simulink library "mDataStoreBlocks_library"  (R2013b)
settings: Solver=ode45  StartTime=0.0  StopTime=10.0  RelTol=1e-3
settings Model: Creator=hungdang  LastModifiedBy=hungdang

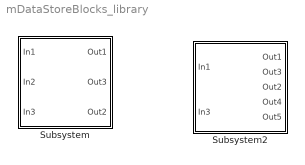
== system mDataStoreBlocks_library ==
  Subsystem : Subsystem  TreatAsAtomicUnit=on
  Subsystem2 : Subsystem  TreatAsAtomicUnit=on
      mask help: This is a simple mask.

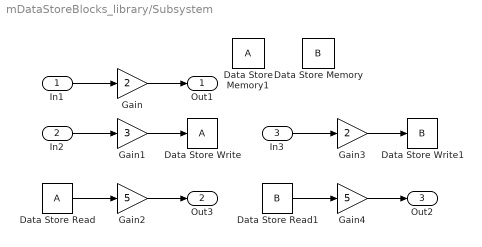
== system mDataStoreBlocks_library/Subsystem ==
  In1 : Inport
  In2 : Inport  Port=2
  In3 : Inport  Port=3
  Data Store Memory : DataStoreMemory  DataStoreName=B  ReadBeforeWriteMsg=warning  WriteAfterWriteMsg=warning  WriteAfterReadMsg=warning
  Data Store Memory1 : DataStoreMemory  ReadBeforeWriteMsg=warning  WriteAfterWriteMsg=warning  WriteAfterReadMsg=warning
  Data Store Read : DataStoreRead
  Data Store Read1 : DataStoreRead  DataStoreName=B
  Data Store Write : DataStoreWrite
  Data Store Write1 : DataStoreWrite  DataStoreName=B
  Gain : Gain  Gain=2
  Gain1 : Gain  Gain=3
  Gain2 : Gain  Gain=5
  Gain3 : Gain  Gain=2
  Gain4 : Gain  Gain=5
  Out1 : Outport
  Out3 : Outport  Port=2
  Out2 : Outport  Port=3
  wires:
  Gain/1 -> Out1/1
  In1/1 -> Gain/1
  Gain1/1 -> Data Store Write/1
  In2/1 -> Gain1/1
  Data Store Read/1 -> Gain2/1
  Gain2/1 -> Out3/1
  Gain3/1 -> Data Store Write1/1
  In3/1 -> Gain3/1
  Data Store Read1/1 -> Gain4/1
  Gain4/1 -> Out2/1

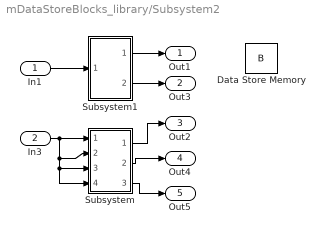
== system mDataStoreBlocks_library/Subsystem2 ==
  In1 : Inport
  In3 : Inport  Port=2
  Data Store Memory : DataStoreMemory  DataStoreName=B  ReadBeforeWriteMsg=warning  WriteAfterWriteMsg=warning  WriteAfterReadMsg=warning
  Subsystem : Subsystem
  Subsystem1 : Subsystem
  Out1 : Outport
  Out3 : Outport  Port=2
  Out2 : Outport  Port=3
  Out4 : Outport  Port=4
  Out5 : Outport  Port=5
  wires:
  Subsystem/3(Out3) -> Out5/1
  Subsystem/2(Out1) -> Out4/1
  Subsystem1/2(Out3) -> Out3/1
  Subsystem1/1(Out1) -> Out1/1
  In1/1 -> Subsystem1/1(In1)
  Subsystem/1(Out2) -> Out2/1
  In3/1 -> Subsystem/1(In3), Subsystem/3(In2), Subsystem/4(In4), Subsystem/2(In1)

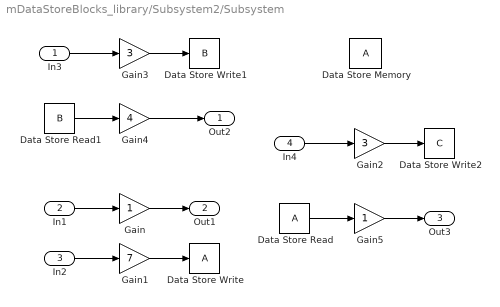
== system mDataStoreBlocks_library/Subsystem2/Subsystem ==
  In3 : Inport
  In1 : Inport  Port=2
  In2 : Inport  Port=3
  In4 : Inport  Port=4
  Data Store Memory : DataStoreMemory  ReadBeforeWriteMsg=warning  WriteAfterWriteMsg=warning  WriteAfterReadMsg=warning
  Data Store Read : DataStoreRead
  Data Store Read1 : DataStoreRead  DataStoreName=B
  Data Store Write : DataStoreWrite
  Data Store Write1 : DataStoreWrite  DataStoreName=B
  Data Store Write2 : DataStoreWrite  DataStoreName=C
  Gain : Gain
  Gain1 : Gain  Gain=7
  Gain2 : Gain  Gain=3
  Gain3 : Gain  Gain=3
  Gain4 : Gain  Gain=4
  Gain5 : Gain
  Out2 : Outport
  Out1 : Outport  Port=2
  Out3 : Outport  Port=3
  wires:
  Gain2/1 -> Data Store Write2/1
  In4/1 -> Gain2/1
  Gain5/1 -> Out3/1
  Data Store Read/1 -> Gain5/1
  In2/1 -> Gain1/1
  Gain1/1 -> Data Store Write/1
  In1/1 -> Gain/1
  Gain/1 -> Out1/1
  Gain3/1 -> Data Store Write1/1
  Data Store Read1/1 -> Gain4/1
  Gain4/1 -> Out2/1
  In3/1 -> Gain3/1

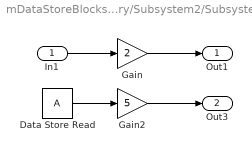
== system mDataStoreBlocks_library/Subsystem2/Subsystem1 ==
  In1 : Inport
  Data Store Read : DataStoreRead
  Gain : Gain  Gain=2
  Gain2 : Gain  Gain=5
  Out1 : Outport
  Out3 : Outport  Port=2
  wires:
  Gain/1 -> Out1/1
  Data Store Read/1 -> Gain2/1
  In1/1 -> Gain/1
  Gain2/1 -> Out3/1
